simulink model "Kalman"  (R2021b)
settings: Solver=VariableStepAuto  StartTime=0.0  StopTime=10.0  RelTol=1e-3
libraries: matrix_library x2
settings Model: Creator=aakas  LastModifiedBy=aakas

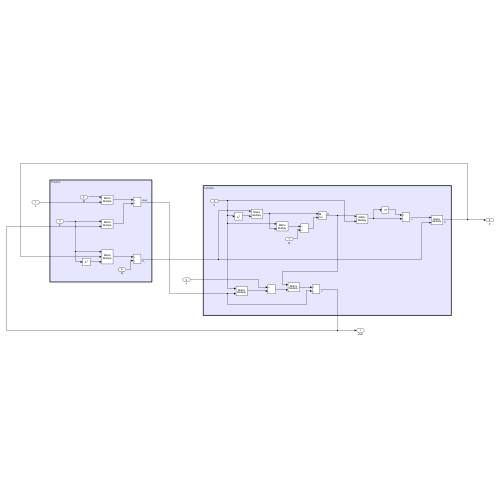
[thumbnail: Simulink's stored preview of the top-level diagram]
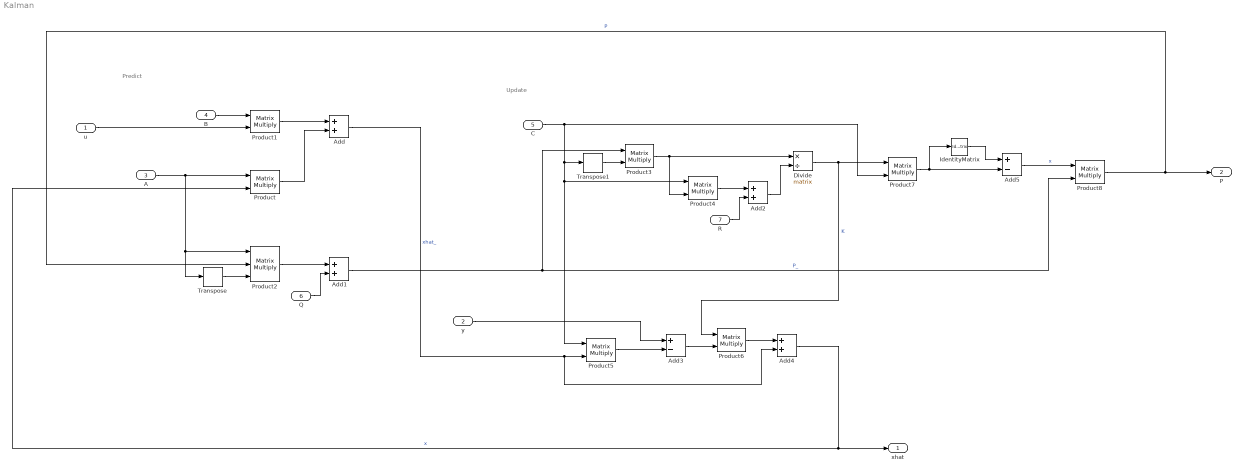
== system Kalman ==
  note: Update
  note: Predict
  u : Inport
  y : Inport  Port=2
  A : Inport  Port=3
  B : Inport  Port=4
  C : Inport  Port=5
  Q : Inport  Port=6
  R : Inport  Port=7
  Add{,1..2,4} (4 alike) : Sum
  Add3 : Sum  Inputs=+-
  Add5 : Sum  Inputs=+-
  Divide : Product  Inputs=*/  Multiplication=Matrix(*)
  IdentityMatrix : IdentityMatrix  InheritOutputPortAttributes=on
  Product{,1,3..8} (8 alike) : Product  Inputs=**  Multiplication=Matrix(*)
  Product2 : Product  Inputs=***  Multiplication=Matrix(*)
  Transpose : matrix_library/Transpose
      settings: SourceProductBaseCode=SL
  Transpose1 : matrix_library/Transpose
      settings: SourceProductBaseCode=SL
  xhat : Outport
  P : Outport  Port=2
  wires:
  u/1 -> Product1/2
  B/1 -> Product1/1
  Transpose/1 -> Product2/3
  Product/1 -> Add/2
  Product1/1 -> Add/1
  Product2/1 -> Add1/1
  Q/1 -> Add1/2
  A/1 -> Product/1, Product2/1, Transpose/1
  Transpose1/1 -> Product3/2
  Product4/1 -> Add2/1
  R/1 -> Add2/2
  Add2/1 -> Divide/2
  Add3/1 -> Product6/2
  Product6/1 -> Add4/1
  Add4/1 -> xhat/1, Product/2  "x"
  IdentityMatrix/1 -> Add5/1
  Product5/1 -> Add3/2
  Add5/1 -> Product8/1  "x"
  y/1 -> Add3/1
  Product3/1 -> Divide/1, Product4/2
  Product8/1 -> P/1, Product2/2  "P"
  Add/1 -> Add4/2, Product5/2  "xhat_"
  Add1/1 -> Product3/1, Product8/2  "P_"
  C/1 -> Product5/1, Product4/1, Transpose1/1, Product7/2
  Divide/1 -> Product7/1, Product6/1  "K"
  Product7/1 -> Add5/2, IdentityMatrix/1
